simulink model "RM3_hwil2c_PI_test_desalv6"  (R2024a)
settings: Solver=ode45  StartTime=0  StopTime=387.2983  FixedStep=0.0005  MaxStep=0.0005  RelTol=1e-3
PreLoadFcn:
  | ng=150;
  | I_cont_design;
  | S_cont_design;
  | Theta_initial=Initial_Angle_Solver(simu_slr,simu_sll,simu_sll);
  | Wave_Analysis_WEC_Sim;
InitFcn:
  | %%% Hydraulic parameters
  | tsim = 1.5;
  | tc = 0.5;
  | Tss = 100e-6;
  | Nseg = 100;
  | Lpipe = 25;
  | Ps_high = 10e5;
  | Ps_low = 0*(Ps_high/3);
  | 
  | %%% Motor parameters
  | Pmax = 15e3;
  | Tmax = 50;
  | Teff = Tmax/2;
  | neff = 1500;
  | wref = 2000*(2*pi/60);
  | 
  | eff = 90;
  | Jmot = 0.005*5;
  | cd = 0.001;
  | kiw = 1e3/10;
  | kpw = 1e3/10;
  | udc = 250;
  | tr = 0.5;
values from neighbouring files (symbols this model uses):
  E_in = 42    [I_cont_design.m]
  In = 8    [I_cont_design.m]
  kii = kci    [I_cont_design.m]
  kis = kcs    [S_cont_design.m]
  kpi = kci/wzi    [I_cont_design.m]
  kps = kcs/wzs    [S_cont_design.m]
  kt = 0.091    [S_cont_design.m]
  La = 1.3e-3    (= 0.0013)    [I_cont_design.m]
  Nn = 4000    [S_cont_design.m]
  Ra = 0.7    [I_cont_design.m]
  simu = simulationClass()    [wecSimInputFile.m]
  simu_sll = 7    [wecSimInputFile.m]
  simu_slr = 1.5    [wecSimInputFile.m]
  T1_s = T1_s-TS    [Wave_Analysis_WEC_Sim.m]
  Ts = simu.dt    [I_cont_design.m]
  waves = waveClass('irregular')    [wecSimInputFile.m]
  wpi = wci*Kboosti    [I_cont_design.m]
  wps = wcs*Kboosts    [S_cont_design.m]
undefined symbols (not defined in the file or in its folder): body, constraint, geometry, hydroData, mooring, pn_flag, pto, T_s, Tf, Tt, Vf, Vfd, X, Y, Z
libraries: nesl_utility x43, fl_lib x25, sm_lib x23, WECSim_Lib_Body_Elements x9, WECSim_Lib_Constraints x5, sh_lib x3, spsMeanLib x2, spsSeriesRLCBranchLib x2, simulink x2, spsVoltageMeasurementLib x2, spsChopperLib x1, slpidlib x1
(part 1 of 5)
Description:
  | Segmented Pipeline Test Rig
  | 
  | The purpose of the rig is to investigate the water hammer effect, which takes place
  | when a variable orifice is abruptly shut off with full flow rate flowing through the
  | branch. The pressure sensor displays pressure at the orifice inlet, while
  | the flow rate meter shows flow rate through the branch. The water hammer-
  | like behavior of the pipeline can be investigated by changing pipeline
  | dimensions, number of segments in the pipeline model, fluid properties, and
  | valve closure speed and value.
  | 
  | 
  | Copyright 2008-2011 The MathWorks, Inc.
settings Model: SimulationMode=accelerator  Creator=MathWorks  LastModifiedBy=jniffene
settings SolverCC: NumberNewtonIterations=2  MaxConsecutiveMinStep=5  ZeroCrossControl=DisableAll  ZeroCrossAlgorithm=Adaptive  AlgebraicLoopSolver=TrustRegion  AutoInsertRateTranBlk=on
settings DataIOCC: LimitDataPoints=on  SaveFormat=Array  SignalLoggingSaveFormat=ModelDataLogs  ReturnWorkspaceOutputs=off
settings OptimizationCC: ExpressionDepthLimit=2147483647  InitFltsAndDblsToZero=on  EfficientMapNaN2IntZero=off  LifeSpan=inf  SimCompilerOptimization=on
settings DebuggingCC: SaveWithParameterizedLinksMsg=none  MergeDetectMultiDrivingBlocksExec=none  SignalResolutionControl=TryResolveAllWithWarning  IgnoredZcDiagnostic=none  SolverPrmCheckMsg=warning  MultiTaskDSMMsg=warning  MultiTaskCondExecSysMsg=none  FcnCallInpInsideContextMsg=warning  UnconnectedInputMsg=warning  UnconnectedOutputMsg=warning  UnconnectedLineMsg=warning  StateNameClashWarn=warning  SFUnexpectedBacktrackingDiag=warning  SFNoUnconditionalDefaultTransitionDiag=warning  ArithmeticOperatorsInVariantConditions=warning
settings HardwareCC: ProdBitPerPointer=32  ProdBitPerSizeT=32  ProdBitPerPtrDiffT=32  ProdLargestAtomicFloat=None  ProdIntDivRoundTo=Undefined  ProdEndianess=Unspecified  ProdWordSize=32  ProdHWDeviceType=32-bit Generic
settings ModelReferenceCC: EnableRefExpFcnMdlSchedulingChecks=on  PropagateSignalLabelsOutOfModel=off
settings SFSimCC: SimUseLocalCustomCode=off  CustomCodeUndefinedFunction=UseInterfaceOnly
settings RTWCC: RTWUseLocalCustomCode=off  GPUComputeCapability=3.5
settings CodeAppCC: StateflowObjectComments=on
settings GRTTargetCC: TargetFcnLib=ansi_tfl_tmw.mat  TargetLangStandard=C89/C90 (ANSI)  CombineOutputUpdateFcns=off  GRTInterface=on
settings ConfigComp: CovMetricSettings=dw  CovSaveCumulativeToWorkspaceVar=on  CovSaveSingleToWorkspaceVar=on  CovExternalEMLEnable=off  CovSFcnEnable=off
settings SimscapeCC: SimscapeNormalizeSystem=off  SimscapeLogType=local  SimscapeLogLimitData=off
settings ExplorerConfigSet: SimMechanicsOpenEditorOnUpdate=off

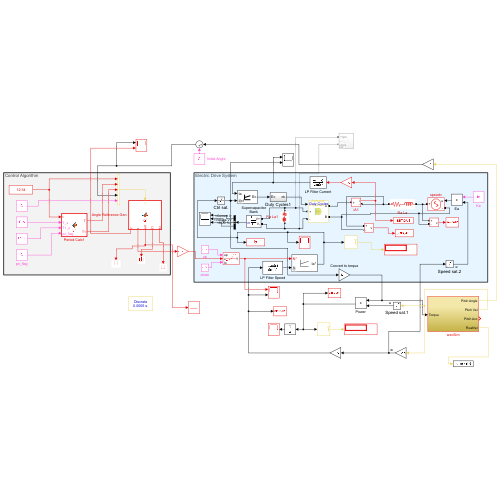
[thumbnail: Simulink's stored preview of the top-level diagram]
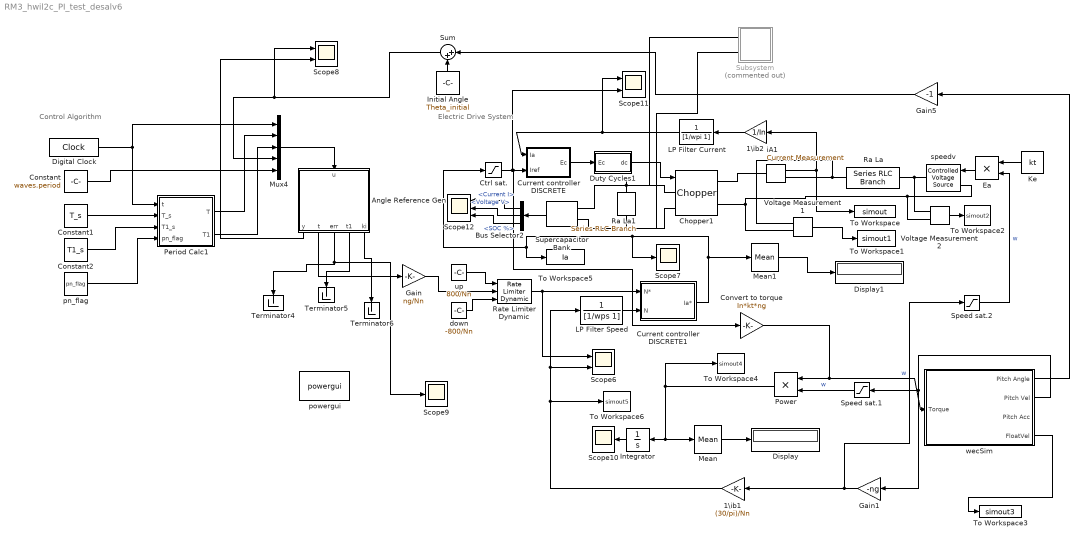
== system RM3_hwil2c_PI_test_desalv6 ==
  note: Electric Drive System
  note: Control Algorithm
  1\ib1 : Gain  Gain=(30/pi)/Nn  SaturateOnIntegerOverflow=on  OutDataTypeStr=Inherit: Same as input  ParamDataTypeStr=Inherit: Same as input
  1\ib2 : Gain  Gain=1/In  SaturateOnIntegerOverflow=on  OutDataTypeStr=Inherit: Same as input  ParamDataTypeStr=Inherit: Same as input
  Angle Reference Gen : MATLAB Function  TreatAsAtomicUnit=on
  Bus Selector2 : BusSelector  OutputSignals=Current I,Voltage V,SOC %
  Chopper1 : spsChopperLib/Chopper  detailLevel=Average  numQuad=4  SnubberResistance=Rsnb  SnubberCapacitance=Csnb  Ron=Ron  ForwardVoltages=[Vf,Vfd]  IGBTParameters=[Tf,Tt]  Ts=simu.dt  converterType=Inverter
      link override Chopper/Average_4q/Bus Selector: OutputSignals=IGBT 1&4
      settings: LibrarySourceBlock=electricdrivelib/Fundamental Drive Blocks/Chopper
  Constant : Constant  Value=waves.period
  Constant1 : Constant  Value=T_s
  Constant2 : Constant  Value=T1_s
  Convert to torque : Gain  Priority=1  Gain=In*kt*ng  SaturateOnIntegerOverflow=on  OutDataTypeStr=Inherit: Same as input  ParamDataTypeStr=Inherit: Same as input
  Ctrl sat. : Saturate  UpperLimit=2  LowerLimit=-2
  Current controller DISCRETE : Subsystem  mask(PI controller){Kp=kpi, Ki=kii, Ts=simu.dt}
      mask prompts: Kp "Proportional gain (Kp)"; Ki "Integral gain (Ki)"; Ts "Sample time (s) :"
      mask help: Proportional-Integral Speed Controller
      mask Display: plot(0,0,100,100,[35,35,65],[70,30,30],[35,65],[45,60])
  Current controller DISCRETE1 : Subsystem  mask(PI controller){Kp=kps*10, Ki=kis/60, Ts=Ts, Kd=0.05*3}
      mask prompts: Kp "Proportional gain (Kp)"; Ki "Integral gain (Ki)"; Ts "Sample time (s) :"; Kd "Differential gain (Kd)"
      mask help: Proportional-Integral Speed Controller
      mask Display: plot(0,0,100,100,[35,35,65],[70,30,30],[35,65],[45,60])
  Digital Clock : DigitalClock  SampleTime=simu.dt
  Display : Display
  Display1 : Display
  Duty Cycles1 : Subsystem
  Ea : Product
  Gain : Gain  Gain=ng/Nn
  Gain1 : Gain  Gain=-ng
  Gain5 : Gain  Gain=-1
  Initial Angle : Constant  Value=Theta_initial
  Integrator : Integrator
  Ke : Constant  Value=kt
  LP Filter Current : TransferFcn  Denominator=[1/wpi 1]
  LP Filter Speed : TransferFcn  Denominator=[1/wps 1]
  Mean : spsMeanLib/Mean  Freq=1/(4*waves.period)  Vinit=0  Ts=0
  Mean1 : spsMeanLib/Mean  Freq=1/(4*waves.period)  Vinit=0  Ts=0
  Mux4 : Mux  Inputs=5
  Period Calc1 : MATLAB Function  TreatAsAtomicUnit=on
  Power : Product
  Ra La : spsSeriesRLCBranchLib/Series RLC Branch  LConnTagsString=__new0  RConnTagsString=__new0  BranchType=RL  Resistance=Ra  Inductance=La  SetiL0=off  InitialCurrent=0  Capacitance=[]  Setx0=off  InitialVoltage=0  Measurements=None
  Ra La1 : spsSeriesRLCBranchLib/Series RLC Branch  LConnTagsString=__new0  RConnTagsString=__new0  BranchType=RL  Resistance=50  Inductance=0  SetiL0=off  InitialCurrent=0  Capacitance=[]  Setx0=off  InitialVoltage=0  Measurements=None
  Rate Limiter Dynamic : simulink/Discontinuities/Rate Limiter Dynamic
  Scope10 : Scope
  Scope11 : Scope  NumInputPorts=2
  Scope12 : Scope  NumInputPorts=3
  Scope6 : Scope  NumInputPorts=2
  Scope7 : Scope
  Scope8 : Scope  NumInputPorts=2
  Scope9 : Scope
  Speed sat.1 : Saturate  UpperLimit=(Nn*pi/30)/ng  LowerLimit=(-Nn*pi/30)/ng
  Speed sat.2 : Saturate  UpperLimit=(Nn*pi/30)  LowerLimit=(-Nn*pi/30)
  Subsystem : Subsystem  Commented=on
  Sum : Sum  Inputs=|++
  Supercapacitor Bank : spsSupercapacitorLib/Supercapacitor  C=100  Rdc=2e-3  Voltage=E_in  Ns=18  Np=1  Vinit=E_in  Temp=25  PresetModel=on  EstParam=off  Nc=1  r=1e-9  epsilon=6.0208e-10  Ich=10  Vstern="[0.161  2.7  7.8]"  Self_dis=on  Ioc=10  Vself="[48  47.8  47.06  44.65]"  demandeplot=off  I="[10  20 100  500]"  Units=sec  Vmax=0  If=0  deltaV=0  alpha=0  sec=0
      settings: LibrarySourceBlock=electricdrivelib/Extra Sources/Supercapacitor
  Terminator4 : Terminator
  Terminator5 : Terminator
  Terminator6 : Terminator
  To Workspace : ToWorkspace  VariableName=simout  SaveFormat=Timeseries  SampleTime=-1
  To Workspace1 : ToWorkspace  VariableName=simout1  SaveFormat=Timeseries  SampleTime=-1
  To Workspace2 : ToWorkspace  VariableName=simout2  SaveFormat=Timeseries  SampleTime=-1
  To Workspace3 : ToWorkspace  VariableName=simout3  SaveFormat=Timeseries  SampleTime=-1
  To Workspace4 : ToWorkspace  VariableName=simout4  SaveFormat=Timeseries  SampleTime=-1
  To Workspace5 : ToWorkspace  VariableName=Ia  SaveFormat=Timeseries  SampleTime=-1
  To Workspace6 : ToWorkspace  VariableName=simout5  SaveFormat=Timeseries  SampleTime=-1
  Voltage Measurement1 : spsVoltageMeasurementLib/Voltage Measurement  Tag=PoWeRsYsTeMmEaSuReMeNt  PhasorSimulation=off  OutputType=Magnitude  PSBequivalent=0
  Voltage Measurement2 : spsVoltageMeasurementLib/Voltage Measurement  Tag=PoWeRsYsTeMmEaSuReMeNt  PhasorSimulation=off  OutputType=Magnitude  PSBequivalent=0
  down : Constant  Value=-800/Nn
  iA1 : spsCurrentMeasurementLib/Current Measurement  PhasorSimulation=off  OutputType=Magnitude  PSBequivalent=0
  pn_flag : Constant  Value=pn_flag
  powergui : sps_lib/powergui  Priority=1  SimulationMode=Discrete  SampleTime=simu.dt  frequency=60  Iterations=50  frequencyindice=0  Pbase=100e6  ErrMax=1e-4  UnitsV=kV  UnitsW=MW  buscounter=0  FunctionMessages=off  echomessages=off  EnableUseOfTLC=off  CurrentSourceSwitches=off  DisableSnubberDevices=off  DisableRonSwitches=off  DisableVfSwitches=off  DisplayEquations=off  AutomaticDiscreteSolvers=off  SolverType=Tustin/Backward Euler (TBE)  Interpol=off  ExternalGateDelay=off  methode=off  Ts=10  x0status=blocks  SPID=off  SwTol=0  HookPort=off  NonlinearTolerance=1e-4  nMaxIteration=100  ContinueOnMaxIteration=off  RestoreLinks=warning  ResistiveCurrentMeasurement=off  Frange=[0:2:500]  Ylog=off  Xlog=on  ShowGrid=off  save=off  variable=ZData  structure=0  ZoomFFT=off  StartTime=0.0  cycles=1  DisplayStyle=1  fundamental=60  FreqAxis=off  MaxFrequency=1000  frequencyindicesteady=1  RmsSteady=1  display=off
  speedv : spsControlledVoltageSourceLib/Controlled Voltage Source  Description=source block  Initialize=on  Source_Type=AC  Amplitude=0  Phase=0  Frequency=0  Measurements=None
  up : Constant  Value=800/Nn
  wecSim : Subsystem
  wires:
  Mean1/1 -> Display1/1
  wecSim/4(FloatVel) -> To Workspace3/1
  Supercapacitor Bank/1 -> Bus Selector2/1
  Bus Selector2/1 -> Scope12/1  "<Current I>"
  iA1/1 -> 1\ib2/1, To Workspace/1
  LP Filter Current/1 -> Scope11/1, Current controller DISCRETE/1(Ia)
  Bus Selector2/3 -> Scope12/3  "<SOC %>"
  Bus Selector2/2 -> Scope12/2  "<Voltage V>"
  1\ib2/1 -> LP Filter Current/1
  wecSim/2(Pitch Vel) -> Speed sat.1/1, Gain1/1
  Angle Reference Gen/3(err) -> Scope9/1, Terminator4/1
  Speed sat.2/1 -> Ea/2  "w"
  1\ib1/1 -> To Workspace6/1, Scope6/2, LP Filter Speed/1
  Current controller DISCRETE/1(Ec) -> Duty Cycles1/1(Ec)
  Power/1 -> To Workspace4/1, Mean/1, Integrator/1
  Voltage Measurement2/1 -> To Workspace2/1
  pn_flag/1 -> Period Calc1/4(pn_flag)
  Duty Cycles1/1(dc) -> Chopper1/1
  Ctrl sat./1 -> Convert to torque/1, Current controller DISCRETE/2(Iref), Scope11/2
  Mean/1 -> Display/1
  Integrator/1 -> Scope10/1
  Current controller DISCRETE1/1(Ia*) -> Mean1/1, Scope7/1, To Workspace5/1, Ctrl sat./1
  Voltage Measurement1/1 -> To Workspace1/1
  Ea/1 -> speedv/1
  Angle Reference Gen/2(t) -> Gain/1
  Ke/1 -> Ea/1
  up/1 -> Rate Limiter Dynamic/1
  Rate Limiter Dynamic/1 -> Scope6/1, Current controller DISCRETE1/1(N*)
  Sum/1 -> Scope8/1, Mux4/4
  Mux4/1 -> Angle Reference Gen/1(u)
  Gain/1 -> Rate Limiter Dynamic/2
  Convert to torque/1 -> wecSim/1(Torque), Power/1
  Period Calc1/1(T) -> Mux4/2
  Gain1/1 -> Speed sat.2/1, 1\ib1/1  "w"
  down/1 -> Rate Limiter Dynamic/3
  LP Filter Speed/1 -> Current controller DISCRETE1/2(N)
  Digital Clock/1 -> Period Calc1/1(t), Mux4/1
  Initial Angle/1 -> Sum/2
  Angle Reference Gen/1(y) -> Scope8/2
  Constant/1 -> Mux4/5
  Angle Reference Gen/4(t1) -> Terminator5/1
  Constant2/1 -> Period Calc1/3(T1_s)
  Gain5/1 -> Sum/1
  Angle Reference Gen/5(ki) -> Terminator6/1
  wecSim/1(Pitch Angle) -> Gain5/1
  Constant1/1 -> Period Calc1/2(T_s)
  Period Calc1/2(T1) -> Mux4/3
  Speed sat.1/1 -> Power/2  "w"
  connections:
  Voltage Measurement1/LConn2 -- speedv/LConn1 -- Voltage Measurement2/LConn2 -- Chopper1/RConn2
  Voltage Measurement2/LConn1 -- Ra La/RConn1 -- speedv/RConn1
  Voltage Measurement1/LConn1 -- Ra La/LConn1 -- iA1/RConn1
  Chopper1/RConn1 -- iA1/LConn1
  Subsystem/LConn2 -- Chopper1/LConn2 -- Ra La1/RConn1 -- Supercapacitor Bank/LConn2
  Subsystem/LConn1 -- Chopper1/LConn1 -- Ra La1/LConn1 -- Supercapacitor Bank/LConn1

== system RM3_hwil2c_PI_test_desalv6/Current controller DISCRETE ==
  Ia : Inport
  Iref : Inport  Port=2
  Ctrl sat. : Saturate  UpperLimit=1  LowerLimit=-1
  Integral gain : Gain  Gain=Ki  SaturateOnIntegerOverflow=on  OutDataTypeStr=Inherit: Same as input  ParamDataTypeStr=Inherit: Same as input
  Integrator : Integrator
  Proportional gain : Gain  Gain=Kp  SaturateOnIntegerOverflow=on  OutDataTypeStr=Inherit: Same as input  ParamDataTypeStr=Inherit: Same as input
  Sum1 : Sum  Inputs=-+  InputSameDT=on  SaturateOnIntegerOverflow=on  OutDataTypeStr=Inherit: Same as first input
  Sum2 : Sum  InputSameDT=on  SaturateOnIntegerOverflow=on  OutDataTypeStr=Inherit: Same as first input
  Ec : Outport  InitialOutput=0
  wires:
  Ctrl sat./1 -> Ec/1
  Sum2/1 -> Ctrl sat./1
  Integrator/1 -> Sum2/2
  Iref/1 -> Sum1/2
  Ia/1 -> Sum1/1
  Sum1/1 -> Proportional gain/1, Integral gain/1
  Integral gain/1 -> Integrator/1
  Proportional gain/1 -> Sum2/1

== system RM3_hwil2c_PI_test_desalv6/Current controller DISCRETE1 ==
  N* : Inport
  N : Inport  Port=2
  Discrete PID Controller : slpidlib/PID Controller  Controller=PID  Form=Parallel  TimeDomain=Continuous-time  UseExternalTs=off  SampleTime=-1  IntegratorMethod=Trapezoidal  FilterMethod=Trapezoidal  ControllerParametersSource=internal  P=Kp  I=Ki  UseKiTs=off  D=Kd  UseExternalDerivativeSource=off  N=100  UseFilter=on  TunerSelectOption=Transfer Function Based (PID Tuner App)  InitialConditionSource=internal  InitialConditionForIntegrator=0  InitialConditionForFilter=0  DifferentiatorICPrevScaledInput=0  ExternalReset=none  TrackingMode=off  Kt=1  LimitOutput=off  SatLimitsSource=internal  UpperSaturationLimit=2  LowerSaturationLimit=-2  LinearizeAsGain=off  AntiWindupMode=none  Kb=1  LimitIntegrator=off  UpperIntegratorSaturationLimit=inf  LowerIntegratorSaturationLimit=-inf  POutMin=[]  POutMax=[]  IOutMin=[]  IOutMax=[]  DOutMin=[]  DOutMax=[]  NOutMin=[]  NOutMax=[]  SumOutMin=[]  SumOutMax=[]  SaturationOutMin=[]  SaturationOutMax=[]  PParamMin=[]  PParamMax=[]  IParamMin=[]  IParamMax=[]  DParamMin=[]  DParamMax=[]  NParamMin=[]  NParamMax=[]  KbParamMin=[]  KbParamMax=[]  KtParamMin=[]  KtParamMax=[]  KbOutMin=[]  KbOutMax=[]  KtOutMin=[]  KtOutMax=[]  IntegratorOutMin=[]  IntegratorOutMax=[]  FilterOutMin=[]  FilterOutMax=[]  SumI1OutMin=[]  SumI1OutMax=[]  SumI2OutMin=[]  SumI2OutMax=[]  SumI3OutMin=[]  SumI3OutMax=[]  SumI4OutMin=[]  SumI4OutMax=[]  SumDOutMin=[]  SumDOutMax=[]  DifferentiatorOutMin=[]  DifferentiatorOutMax=[]  FilterDiffOutCoefMin=[]  FilterDiffOutCoefMax=[]  ReciprocalOutMin=[]  ReciprocalOutMax=[]  SumDenOutMin=[]  SumDenOutMax=[]  SumNumOutMin=[]  SumNumOutMax=[]  DivideOutMin=[]  DivideOutMax=[]  UdiffTsProdOutMin=[]  UdiffTsProdOutMax=[]  NTsProdOutMin=[]  NTsProdOutMax=[]  UintegralTsProdOutMin=[]  UintegralTsProdOutMax=[]  UngainTsProdOutMin=[]  UngainTsProdOutMax=[]  ClampingZeroOutDataTypeStr=Inherit: Inherit via back propagation  ClampingZeroOutMin=[]  ClampingZeroOutMax=[]  FilterDenConstantOutDataTypeStr=Inherit: Inherit via back propagation  FilterDenConstantOutMin=[]  FilterDenConstantOutMax=[]  PCopyOutDataTypeStr=Inherit: Inherit via back propagation  PCopyOutMin=[]  PCopyOutMax=[]  NCopyOutDataTypeStr=Inherit: Inherit via back propagation  NCopyOutMin=[]  NCopyOutMax=[]  IntegratorContinuousStateAttributes=''  IntegratorStateMustResolveToSignalObject=off  IntegratorRTWStateStorageClass=Auto  FilterContinuousStateAttributes=''  FilterStateMustResolveToSignalObject=off  FilterRTWStateStorageClass=Auto  ParallelPVariant=InternalParameters  IdealPVariant=Disabled  IVariant=InternalParameters  DVariant=InternalParameters  IntegratorVariant=Continuous  SatVariant=Disabled  AWVariant=Passthrough  PCopyVariant=Disabled  TRVariant=Disabled  FdbkBlocksVariant=Forward  IdealPFdbkVariant=Disabled  SatFdbkVariant=Disabled  DerivativeFilterVariant=ContFilter  NVariant=InternalParameters  NCopyVariant=Disabled  FilterICVariant=InternalICsFilter  IntegratorICVariant=InternalICs  ExternalResetVariant=Disabled  TRSumVariant=Passthrough  SumFdbkVariant=Disabled  SumVariant=Sum_PID  TsampFilterVariant=InternalTs  TsampNgainVariant=Passthrough  TsampIntegralVariant=Disabled_SignalSpec  ExternalSaturationOutDataTypeStr=Inherit: Same as second input  DerivativeSourceVariant=ErrorSignal
  Sum1 : Sum  Inputs=+-  InputSameDT=on  SaturateOnIntegerOverflow=on  OutDataTypeStr=Inherit: Same as first input
  Ia* : Outport  InitialOutput=0
  wires:
  Discrete PID Controller/1 -> Ia*/1
  N/1 -> Sum1/2
  N*/1 -> Sum1/1
  Sum1/1 -> Discrete PID Controller/1

== system RM3_hwil2c_PI_test_desalv6/Duty Cycles1 ==
  Ec : Inport
  Add : Sum  Inputs=+-
  Bus Creator2 : BusCreator  Inputs=2
  Constant : Constant
  Duty Cycle : Fcn  Expr=0.5*(u[1]+1)
  dc : Outport
  wires:
  Bus Creator2/1 -> dc/1
  Ec/1 -> Duty Cycle/1
  Constant/1 -> Add/1
  Duty Cycle/1 -> Add/2, Bus Creator2/1  "IGBT 1&4"
  Add/1 -> Bus Creator2/2  "IGBT 2&3"

== system RM3_hwil2c_PI_test_desalv6/Subsystem ==
  note: Copyright 2016 - 2020 MathWorks AB
  "Brine " : fl_lib/Hydraulic/Hydraulic Elements/Hydraulic Reference
  Clock1 : Clock
  Current-Voltage Simscape Interface : spsCurrentVoltageSimscapeInterfaceLib/Current-Voltage Simscape Interface  DFT=on  FMode=Low pass filter (continuous)  T=1e-6  Ts=50e-6  i0=0  v0=E_in  Sd=Specialized Power Systems side  Measurements=off
      settings: LibrarySourceBlock=|
      | sps_lib/Utilities/Current-Voltage
      | Simscape Interface
  Electrical Reference : fl_lib/Electrical/Electrical Elements/Electrical Reference
  Fixed-Displacement Pump : sh_lib/Pumps and Motors/Fixed-Displacement Pump  D=(5e-6)/100 m^3/rad  loss_spec=1  w_nominal=188 rad/s  pr_nominal=100e5 Pa  visc_nominal=18 cSt  dens_nominal=984.328 kg/m^3  efficiency_vol=1  no_load_torque=0 N*m  torque_pressure_coeff=1*(5e-6)*((1)/(1)-1 ) N*m/Pa  p_diff_eff_TLU=[100000.0, 1000000.0, 2000000.0] Pa  omega_eff_TLU=[25.0, 50.0, 100.0, 200.0, 300.0, 400.0] rad/s  vol_eff_TLU=[0.816, 0.908, 0.954, 0.977, 0.981, 0.984; 0.325, 0.663, 0.831, 0.916, 0.925, 0.946; 0.137, 0.568, 0.78, 0.892, 0.893, 0.91]  mech_eff_TLU=[0.996, 0.996, 0.996, 0.996, 0.996, 0.996; 0.988, 0.989, 0.989, 0.989, 0.989, 0.99; 0.981, 0.981, 0.982, 0.982, 0.983, 0.984]  p_diff_loss_TLU=[100000.0, 1000000.0, 2000000.0] Pa  omega_loss_TLU=[25.0, 50.0, 100.0, 200.0, 300.0, 400.0] rad/s  vol_loss_TLU=[0.023, 0.023, 0.023, 0.023, 0.0285, 0.032; 0.0844, 0.0842, 0.0845, 0.084, 0.1125, 0.108; 0.1079, 0.108, 0.11, 0.108, 0.1605, 0.18] * 1e-3 m^3/s  mech_loss_TLU=[0.002, 0.002, 0.002, 0.002, 0.002, 0.002; 0.0607, 0.0556, 0.0556, 0.0556, 0.0556, 0.0505; 0.1937, 0.1937, 0.1833, 0.1833, 0.1729, 0.1626] N*m  pressure_threshold=1e5 Pa  omega_threshold=10 rad/s  quadrant_check=0  pressure_check=0  min_valid_pressure=0 Pa  vol_eff_min=1e-3  vol_eff_max=1  mech_eff_min=1e-3  mech_eff_max=1
      settings: InternalSimscapePortConfiguration="{\"Bottom\":[],\"Left\":[{\"id\":\"S\",\"label\":\"S\",\"type\":\"foundation.mechanical.rotational.rotational\"}],\"Right\":[{\"id\":\"P\",\"label\":\"P\",\"type\":\"foundation.hydraulic.hydraulic\"},{\"id\":\"T\",\"label\":\"T\",\"type\":\"foundation.hydraulic.hydraulic\"}],\"Top\":[]}"
  HR2 : fl_lib/Hydraulic/Hydraulic Elements/Hydraulic Reference  Tag=Factory Generic
  Hydraulic Fluid : sh_lib/Hydraulic Utilities/Hydraulic Fluid  Tag=Factory Generic  SelFluid=24  SysTemp=60  TrapAir=0.001  ViscDerFactor=1  range_error=2
  Logging : Subsystem
  Mechanical Rotational Reference : fl_lib/Mechanical/Rotational Elements/Mechanical Rotational Reference
  Motor : ee_lib/Electromechanical/Motor & Drive (System Level)  torque_speed_param=2  overtorque_param=ee.enum.electromech.overtorque.no  T_t=[0.09 0.08 0.07 0] N*m  T_t_intermittent=[.36, .32, .28, 0] N*m  T_t_2D=[.09, .09, .09; .08, .08, .08; .07, .07, .07; 0, 0, 0] N*m  T_t_intermittent_2D=[.36, .36, .36; .32, .32, .32; .28, .28, .28; 0, 0, 0] N*m  w_t=[ 0 3.75e+3 7.5e+3 8e+3 ] rpm  vdc_t=[6, 12, 24] V  torque_max=5 N*m  power_max=100 W  torque_max_intermittent=0.4 N*m  power_max_intermittent=120 W  time_overtorque=30 s  time_recover=60 s  Tc=0.05 s  EnableSwitch=simscape.enum.onoff.off  losses_param=1  eff=eff  w_eff=neff rpm  T_eff=Teff N*m  Piron=0 W  Pbase=0 W  w_eff_vec=[-8000 -4000 0 4000 8000] rpm  T_eff_vec=[0 0.03 0.06 0.09] N*m  v_eff_vec=[100, 250, 400] V  losses_mat=[1.49 1.67 2.21 3.10; 0.42 0.69 1.14 2.03; 0.06 0.24 0.78 1.68; 0.42 0.69 1.14 2.03; 1.49 1.67 2.21 3.10] W  efficiency_mat=[95, 95, 95, 95; 95, 95, 95, 95; 95, 95, 95, 95; 95, 95, 95, 95; 95, 95, 95, 95]  losses_mat_3D=ones(5, 4, 3) W  efficiency_mat_3D=95 * ones(5, 4, 3)  Res=0 Ohm  enable_fault=simscape.enum.onoff.off  fault_condition=1  fault_threshold=0.5  J=4.2e-4 kg*m^2  lam=1.5e-4 N*m/(rad/s)  speed0=0 rpm  faulted_specify=off  faulted_priority=None  faulted=0  faulted_nominal_specify=off  faulted_nominal_value=1  faulted_nominal_unit=1  isSwitchedOff_specify=off  isSwitchedOff_priority=None  isSwitchedOff=0  isSwitchedOff_nominal_specify=off  isSwitchedOff_nominal_value=1  isSwitchedOff_nominal_unit=1  torqueLimitContinuous_specify=off  torqueLimitContinuous_priority=None  torqueLimitContinuous=0 N*m  torqueLimitContinuous_nominal_specify=off  torqueLimitContinuous_nominal_value=1  torqueLimitContinuous_nominal_unit=N*m  alpha=3.93e-3 1/K  Tmeas=25 degC  Tmeas2=125 degC  losses_mat_T2=[1.49, 1.74, 2.49, 3.74; .42, .67, 1.42, 2.67; .06, .31, 1.06, 2.31; .42, .67, 1.42, 2.67; 1.49, 1.74, 2.49, 3.74] W  efficiency_mat_T2=[95, 95, 95, 95; 95, 95, 95, 95; 95, 95, 95, 95; 95, 95, 95, 95; 95, 95, 95, 95]  losses_mat_3D_T2=ones(5, 4, 3) W  efficiency_mat_3D_T2=95 * ones(5, 4, 3)  thermal_mass=100 J/K  initial_temperature=25 degC
      settings: LogSimulationData=on
  Permeate : fl_lib/Hydraulic/Hydraulic Elements/Hydraulic Reference
  Q_sensor_vfd : Subsystem
  RO Membrane : Subsystem
      mask Display: image('/Users/yyu/Dropbox/WorksNREL/ResearchWork/Desalination/JSME Runs/Images/ReverseOsmosisMembrane.jpg');
  Sensor : Subsystem
  Sensor Mec (VFD) : Subsystem
  Simulink-PS Converter1 : nesl_utility/Simulink-PS Converter  PhysicalDomain=network_engine_domain  SubClassName=ps_input  LeftPortType=input  RightPortType=output  PseudoPeriodic=off  Frequencies=[]  NoiseDistribution=none  NoiseParameters=[]  Unit=rad/s  AffineConversion=off  FilteringAndDerivatives=zero  SimscapeFilterOrder=1  InputFilterTimeConstant=.001  UdotUserProvided=1
  Solver Configuration : nesl_utility/Solver Configuration  PhysicalDomain=network_engine_domain  SubClassName=solver  LeftPortType=input  RightPortType=generic  Tones=[]  Harmonics=[]  SimulateNoise=off  Profile=off  UseLocalSampling=off  EnableSwitchedLinearOptims=on  FrequencyDomain=off  UseCCode=off  RelTol=0.001  AbsTol=1e-06  MinStep=1e-09  ToWorkspace=off  RevertToSquareIcSolve=off  NumHomotopyIterations=100  PhasorMode=off  PhasorModeNumHarmonics=1  ConsistencySolver=NEWTON_FTOL  IndexReductionMethod=DerivativeReplacement  DoDC=off  ResidualTolerance=1e-9  ConsistencyTolSource=GLOBAL  ConsistencyAbsTol=0.001  ConsistencyRelTol=0.001  ConsistencyTolFactor=0.001  UseLocalSolver=off  LocalSolverChoice=NE_BACKWARD_EULER_ADVANCER  ResolveIndetEquations=on  FunctionEvalNumThread=1  LocalSolverSampleTime=Tss  DoFixedCost=off  MaxNonlinIter=3  MaxModeIter=2  ComputeImpulses=off  ImpulseIterations=2  LinearAlgebra=Sparse  LinearAlgebraNumThread=0  EquationFormulation=NE_TIME_EF  DelaysMemoryBudget=1024  AutomaticFiltering=on  FilteringTimeConstant=0.001  PartitionStorageMethod=AS_NEEDED  PartitionMemoryBudget=1024  PartitionMethod=FAST  MultibodyUseLocalSolver=off  MultibodyLocalSolverChoice=ODE1  MultibodyLocalSolverSampleTime=0.001
  Speed control : Subsystem
  speed profile : Lookup_n-D  NumberOfTableDimensions=1  BreakpointsForDimension1=[0 10 20]  Table=[0 1 1]*1.122790000000000e+02  InternalRulePriority=Speed  RndMeth=Simplest
  +sps : PMIOPort  Side=Left
  -sps : PMIOPort  Port=2  Side=Left
  wires:
  Clock1/1 -> speed profile/1
  speed profile/1 -> Simulink-PS Converter1/1
  connections:
  Electrical Reference/LConn1 -- Current-Voltage Simscape Interface/RConn2 -- Motor/RConn1
  Fixed-Displacement Pump/LConn1 -- Sensor Mec (VFD)/RConn1
  "Brine "/LConn1 -- RO Membrane/RConn2
  Solver Configuration/RConn1 -- Fixed-Displacement Pump/RConn1 -- Hydraulic Fluid/RConn1 -- Q_sensor_vfd/LConn1
  Simulink-PS Converter1/RConn1 -- Speed control/LConn1
  Speed control/RConn1 -- Motor/LConn2
  Motor/RConn2 -- Speed control/LConn2
  Permeate/LConn1 -- RO Membrane/RConn1
  Current-Voltage Simscape Interface/RConn1 -- Sensor/LConn1
  Q_sensor_vfd/RConn1 -- RO Membrane/LConn1
  Sensor/RConn1 -- Motor/LConn1
  Motor/LConn3 -- Sensor Mec (VFD)/LConn1
  Fixed-Displacement Pump/RConn2 -- HR2/LConn1
  Motor/RConn3 -- Mechanical Rotational Reference/LConn1
  Current-Voltage Simscape Interface/LConn2 -- -sps/RConn1
  Current-Voltage Simscape Interface/LConn1 -- +sps/RConn1

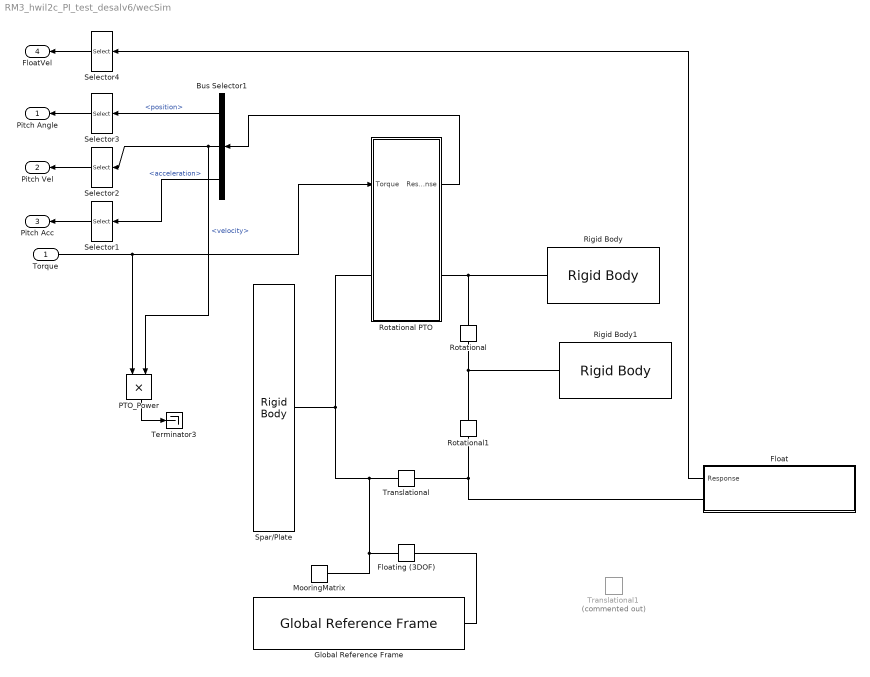
== system RM3_hwil2c_PI_test_desalv6/wecSim ==
  Torque : Inport
  Bus Selector1 : BusSelector  OutputSignals=position,velocity,acceleration
  Float : Subsystem  AncestorBlock=WECSim_Lib_Body_Elements/Rigid Body  Variant=on  AllowZeroVariantControls=on  mask(Rigid Body){body=body(1), InputFileText=Global Reference Frame option "Use Input File" is selected., h5File=hydroData/*.h5, geometryFile=geometry/*.stl, mass=0, inertia=0 0 0, inertiaProducts=0 0 0, nonHydro=0, nonlinearHydro=0, centerGravity=0 0 0, centerBuoyancy=0 0 0, dof=6, volume=0, QTFs=0, flex=0, displacement=0 0 0, axis=0 1 0, angle=0, option=0, cd=0 0 0, ca=0 0 0, area=0 0 0, VME=0, rgME=0 0 0, z=0 0 1}
      mask prompts: body "Body Number:"; mass "Body Mass [kg]:"; inertia "MoI [kg*m^2]:"; inertiaProducts "Product of Inertia [kg*m^2]"; nonHydro "Nonhydro Body"; nonlinearHydro "Nonlinear Hydrodynamics"; centerGravity "Center of gravity [m]"; centerBuoyancy "Center of buoyancy [m]"; dof "Degrees of freedom"; volume "Displaced Volume [m^3]"; flex "Flexible Body"; displacement "Initial Linear Displacement"; axis "Initial Angular Displacement Axis"; angle "Initial Angular Displacement"; option "On/Off"; cd "Drag coefficient"; ca "Added mass coefficient"; area "Characteristic Area"; VME "Characteristic Volume"; rgME "Point of Application"; z "Z axis"
      mask help:
      | A rigid body has no generalized body modes. It can be a standard hydrodynamic body, a drag body, or a non-hydrodynamic body.
      |
      | The variable name input below must be 'body(i)' where i=1,2,...
      | body(i) must be defined in the input file with the fields appropriate to each variant.
      mask init:
      | if exist('body','var')
      |     %%
      |     % Hydro Body
      |     h = [gcb '/Hydrodynamic Body'];
      |     responseName = ['sv_b' num2str(body.number) '_hydroBody'];
      |     set_param(h,'VariantControl',responseName);
      |     %%
      |     % Hydro Body Morison Element: Off
      |     h = [gcb '/Hydrodynamic Body/Morison Element and Viscous Damping Force Calculation/Morison Element Variant Subsystem/Morison Element Off'];
      |     responseName = ['sv_b' num2str(body.number) '_MEOff'];
      |     set_param(h,'VariantControl',responseName);
      |     %%
      |     % Hydro Body Morison Element: On
      |     h = [gcb '/Hydrodynamic Body/Morison Element and Viscous Damping Force Calculation/Morison Element Variant Subsystem/Morison Element On'];
      |     responseName = ['sv_b' num2str(body.number) '_MEOn'];
      |     set_param(h,'VariantControl',responseName);
      |     %%
      |     % Hydro Body Nonlinear Froude Krylov Force: Off
      |     h = [gcb '/Hydrodynamic Body/Wave Diffraction and Excitation Force Calculation/Nonlinear FK Force Variant Subsystem/No Nonlinear FroudeKrylov Force'];
      |     responseName = ['sv_b' num2str(body.number) '_linearHydro'];
      |     set_param(h,'VariantControl',responseName);
      |     %%
      |     % Hydro Body Nonlinear Froude Krylov Force: On
      |     h = [gcb '/Hydrodynamic Body/Wave Diffraction and Excitation Force Calculation/Nonlinear FK Force Variant Subsystem/With Nonlinear FroudeKrylov Force'];
      |     responseName = ['sv_b' num2str(body.number) '_nonlinearHydro'];
      |     set_param(h,'VariantControl',responseName);
      |     %%
      |     % Hydro Body Nonlinear Restoring: Off
      |     h = [gcb '/Hydrodynamic Body/Hydrostatic Restoring Force Calculation/Linear and Nonlinear Restoring Force Variant Subsystem/Linear Hydrostatic Restoring Force'];
      |     responseName = ['sv_b' num2str(body.number) '_linearHydro'];
      |     set_param(h,'VariantControl',responseName);
      |     %%
      |     % Hydro Body Nonlinear Restoring: On
      |     h = [gcb '/Hydrodynamic Body/Hydrostatic Restoring Force Calculation/Linear and Nonlinear Restoring Force Variant Subsystem/Nonlinear Hydrostatic Restoring Force'];
      |     responseName = ['sv_b' num2str(body.number) '_nonlinearHydro'];
      |     set_param(h,'VariantControl',responseName);
      |     %%
      |     % Hydro Body Regular Excitation Passive Yaw: Off
      |     h = [gcb '/Hydrodynamic Body/Wave Diffraction and Excitation Force Calculation/Linear Wave Excitation Force Variant Subsystem/Regular Wave ' newline 'Excitation Force'];
      |     responseName = ['sv_regularWaves_b' num2str(body.number)];
      |     set_param(h,'VariantControl',responseName);
      |     %%
      |     % Hydro Body Regular Excitation Passive Yaw: On
      |     h = [gcb '/Hydrodynamic Body/Wave Diffraction and Excitation Force Calculation/Linear Wave Excitation Force Variant Subsystem/Regular Wave ' newline 'NonLinear Yaw'];
      |     responseName = ['sv_regularWavesYaw_b' num2str(body.number)];
      |     set_param(h,'VariantControl',responseName);
      |     %%    
      |     % Hydro Body Irregular Excitation Passive Yaw: Off
      |     h = [gcb '/Hydrodynamic Body/Wave Diffraction and Excitation Force Calculation/Linear Wave Excitation Force Variant Subsystem/Irregular Wave ' newline 'Excitation Force'];
      |     responseName = ['sv_irregularWaves_b' num2str(body.number)];
      |     set_param(h,'VariantControl',responseName);
      |     %%
      |     % Hydro Body Irregular Excitation Passive Yaw: On
      |     h = [gcb '/Hydrodynamic Body/Wave Diffraction and Excitation Force Calculation/Linear Wave Excitation Force Variant Subsystem/Irregular Wave ' newline 'NonLinearYaw'];
      |     responseName = ['sv_irregularWavesYaw_b' num2str(body.number)];
      |     set_param(h,'VariantControl',responseName);
      |     %%
      |     % Hydro Body Nonlinear Froude Krylov or Restoring: Instantaneous Free Surface
      |     h = [gcb '/Hydrodynamic Body/Nonlinear Wave Elevation/Linear or Instantaneous Free Surface/Instantaneous Water Free Surface'];
      |     responseName = ['sv_b' num2str(body.number) '_instFS'];
      |     set_param(h,'VariantControl',responseName);
      |     %%
      |     % Hydro Body Nonlinear Froude Krylov or Restoring: Mean Free Surface
      |     h = [gcb '/Hydrodynamic Body/Nonlinear Wave Elevation/Linear or Instantaneous Free Surface/Mean Water Free Surface'];
      |     responseName = ['sv_b' num2str(body.number) '_meanFS'];
      |     set_param(h,'VariantControl',responseName);
      |     %% Variable hydro on/off
      |     % Variable hydro control - variable hydro off
      |     h = [gcb '/Hydrodynamic Body/Variable Hydrodynamics Control/Variable Hydrodynamics Subsystem/noVariableHydro'];
      |     responseName = ['sv_b' num2str(body.number) '_noVariableHydro'];
      |     set_param(h,'VariantControl',responseName);
      |     % Variable hydro control - variable hydro on
      |     h = [gcb '/Hydrodynamic Body/Variable Hydrodynamics Control/Variable Hydrodynamics Subsystem/variableHydro'];
      |     responseName = ['sv_b' num2str(body.number) '_variableHydro'];
      |     set_param(h,'VariantControl',responseName);
      |     % CIC - variable hydro off
      |     h = [gcb '/Hydrodynamic Body/Wave Radiation Forces Calculation/SS CI and Constant-Damping-CoeVariant Subsystem/Convolution Integral Calculation/Convolution Variant Subsystem/Convolution Integral Calculation'];
      |     responseName = ['sv_b' num2str(body.number) '_noVariableHydro'];
      |     set_param(h,'VariantControl',responseName);
      |     % CIC - variable hydro on
      |     h = [gcb '/Hydrodynamic Body/Wave Radiation Forces Calculation/SS CI and Constant-Damping-CoeVariant Subsystem/Convolution Integral Calculation/Convolution Variant Subsystem/Convolution Integral Surface Calculation'];
      |     responseName = ['sv_b' num2str(body.number) '_variableHydro'];
      |     set_param(h,'VariantControl',responseName);
      |     %%
      |     % Non-Hydro Body
      |     h = [gcb '/Non-Hydro Body'];
      |     responseName = ['sv_b' num2str(body.number) '_nonHydroBody'];
      |     set_param(h,'VariantControl',responseName);
      |     %%
      |     % Drag Body
      |     h = [gcb '/Drag Body'];
      |     responseName = ['sv_b' num2str(body.number) '_dragBody'];
      |     set_param(h,'VariantControl',responseName);
      |     %%
      |     % Drag Body Morison Element: Off
      |     h = [gcb '/Drag Body/Morison Element and Viscous Damping Force Calculation/Morison Element Variant Subsystem/Morison Element Off'];
      |     responseName = ['sv_b' num2str(body.number) '_MEOff'];
      |     set_param(h,'VariantControl',responseName);
      |     %%
      |     % Drag Body Morison Element: On
      |     h = [gcb '/Drag Body/Morison Element and Viscous Damping Force Calculation/Morison Element Variant Subsystem/Morison Element On'];
      |     responseName = ['sv_b' num2str(body.number) '_MEOn'];
      |     set_param(h,'VariantControl',responseName);
      |     %% 
      |     % Hydro Body QTF: Off
      |     h = [gcb '/Hydrodynamic Body/Wave Diffraction and Excitation Force Calculation/Second Order Excitation Force Variant Subsystem/No Second Order Excitation Force'];
      |     responseName = ['sv_b' num2str(body.number) '_noSecondOrderExt'];
      |     set_param(h,'VariantControl',responseName);
      |     %%
      |     % Hydro Body QTF: On
      |     h = [gcb '/Hydrodynamic Body/Wave Diffraction and Excitation Force Calculation/Second Order Excitation Force Variant Subsystem/With Second Order Excitation Force'];
      |     responseName = ['sv_b' num2str(body.number) '_secondOrderExt'];
      |     set_param(h,'VariantControl',responseName);
      |     %%
      |     % Set zero active variant controls to prevent label issue
      |     set_param(gcb,'AllowZeroVariantControls','on');
      | end
      | clear bc h geomFile responseName
      settings: AttributesFormatString=%<body>
      mask Help:
      | A rigid body has no generalized body modes. It can be a standard hydrodynamic body, a drag body, or a non-hydrodynamic body.
      | 
      | The variable name input below must be 'body(i)' where i=1,2,...
      | body(i) must be defined in the input file with the fields appropriate to each variant.
      mask TypeOptions nonHydro: 0 | 1 | 2
      mask Callback nonHydro: bodyClassCallback(gcbh)
      mask TypeOptions nonlinearHydro: 0 | 1 | 2
      mask TypeOptions QTFs: 0 | 1 | 2
      mask TypeOptions flex: 0 | 1
      mask TypeOptions option: 0 | 1 | 2
      mask Callback option: bodyClassCallback(gcbh)
      mask DialogControl CustomParameterGroup Prompt: Custom Parameters
      mask DialogControl std_opts Prompt: Standard Options
      mask DialogControl H5button Prompt: Select .h5 File
      mask DialogControl H5button Callback: h5ButtonCallback(gcbh)
      mask DialogControl STLbutton Prompt: Select .stl File
      mask DialogControl STLbutton Callback: stlButtonCallback(gcbh)
      mask DialogControl inertia Tooltip: Moment of Inertia
      mask DialogControl inertiaProducts Tooltip: Product of Inertia (Ixy, Ixz, Iyz)
      mask DialogControl initial Prompt: Initial Displacement
      mask DialogControl morisonElement Prompt: Morison Element
      mask DialogControl rgME Tooltip: The vector from the body COG to point of application for the Morison Element
      mask DialogControl z Tooltip: The unit normal vector center axis of the Morison Element
  Floating (3DOF) : WECSim_Lib_Constraints/Floating (3DOF)  constraint=constraint(1)  loc="0  0  0"  displacement=0 0 0  y=0 1 0  z=0 0 1  upperLimitSpecify=off  upperLimitBound=0  upperLimitTransitionRegionWidth=0  upperLimitStiffness=0  upperLimitDamping=0  lowerLimitSpecify=off  lowerLimitBound=0  lowerLimitTransitionRegionWidth=0  lowerLimitStiffness=0  lowerLimitDamping=0
      settings: AttributesFormatString=%<constraint>  SourceProductName=WEC-Sim
  Global Reference Frame : WECSim_Lib_Frames/Global Reference Frame  waves=waves  simu=simu  InputMethod=Input File  InputFile=wecSimInputFile.m  mode=normal  explorer=off  solver=ode4  startTime=0  rampTime=100  endTime=400  dt=0.1  cicEndTime=60  stateSpace=0  WaveClass=regular  height=2.5  period=8  elevationFile=NOT DEFINED  spectrumFile=NOT DEFINED  direction=0  spread=1  spectrumType=NOT DEFINED  phaseSeed=0  option=EqualEnergy
  MooringMatrix : WECSim_Lib_Moorings/MooringMatrix  mooring=mooring(1)  loc=0 0 0  preTension=[0 0 0 0 0 0]  stiffness={ '0', '0', '0', '0', '0', '0'; '0', '0', '0', '0', '0', '0'; '0', '0', '0', '0', '0', '0'; '0', '0', '0', '0', '0', '0'; '0', '0', '0', '0', '0', '0'; '0', '0', '0', '0', '0', '0' }  damping={ '0', '0', '0', '0', '0', '0'; '0', '0', '0', '0', '0', '0'; '0', '0', '0', '0', '0', '0'; '0', '0', '0', '0', '0', '0'; '0', '0', '0', '0', '0', '0'; '0', '0', '0', '0', '0', '0' }
      settings: AttributesFormatString=%<mooring>  SourceProductName=WEC-Sim
  PTO_Power : Product  Inputs=**
  Rigid Body : WECSim_Lib_Body_Elements/Rigid Body  body=body(3)  h5File=hydroData/*.h5  geometryFile=geometry/*.stl  mass=0  inertia=0 0 0  inertiaProducts=0 0 0  nonHydro=0  nonlinearHydro=0  centerGravity=0 0 0  centerBuoyancy=0 0 0  dof=6  volume=0  QTFs=0  displacement=0 0 0  axis=0 1 0  angle=0  option=0  cd=0 0 0  ca=0 0 0  area=0 0 0  VME=0  rgME=0 0 0  z=0 0 1
      link override Non-Hydro Body/Mass: Value=body.mass
  Rigid Body1 : WECSim_Lib_Body_Elements/Rigid Body  body=body(4)  h5File=hydroData/*.h5  geometryFile=geometry/*.stl  mass=0  inertia=0 0 0  inertiaProducts=0 0 0  nonHydro=0  nonlinearHydro=0  centerGravity=0 0 0  centerBuoyancy=0 0 0  dof=6  volume=0  QTFs=0  displacement=0 0 0  axis=0 1 0  angle=0  option=0  cd=0 0 0  ca=0 0 0  area=0 0 0  VME=0  rgME=0 0 0  z=0 0 1
      link override Non-Hydro Body/Mass: Value=body.mass
  Rotational : WECSim_Lib_Constraints/Rotational  constraint=constraint(3)  loc="0  0  0"  displacement=0 0 0  y=0 1 0  z=0 0 1  upperLimitSpecify=off  upperLimitBound=0  upperLimitTransitionRegionWidth=0  upperLimitStiffness=0  upperLimitDamping=0  lowerLimitSpecify=off  lowerLimitBound=0  lowerLimitTransitionRegionWidth=0  lowerLimitStiffness=0  lowerLimitDamping=0
      settings: AttributesFormatString=%<constraint>
  Rotational PTO : Subsystem  AncestorBlock=WECSim_Lib_PTOs/Rotational PTO  mask(PTO){pto=pto(1), InputFileText=Global Reference Frame option "Use Input File" is selected., loc=0  0  0, stiffness=0, damping=0, equilibriumPosition=0, pretension=0, displacement=0 0 0, x=, y=0 1 0, z=0 0 1, upperLimitSpecify=off, upperLimitBound=0, upperLimitTransitionRegionWidth=0, upperLimitStiffness=0, upperLimitDamping=0, lowerLimitSpecify=off, lowerLimitBound=0, lowerLimitTransitionRegionWidth=0, lowerLimitStiffness=0, lowerLimitDamping=0}
      mask prompts: pto "PTO Name:"; loc "Location [m]:"; stiffness "Stiffness [N/m]:"; damping "Damping [N/(m/s)]:"; equilibriumPosition "Equilibrium position [m, deg]:"; pretension "Pretension [N, Nm]:"; displacement "Initial linear displacement [m]:"; x "X-axis [m]:"; y "Y-axis [m]:"; z "Z-axis [m]:"; upperLimitSpecify "Upper limit"; upperLimitBound "Upper limit bound [m, deg]:"; upperLimitTransitionRegionWidth "Upper limit transition region width [m, deg]:"; upperLimitStiffness "Upper limit stiffness [N/m, Nm/rad]:"; upperLimitDamping "Upper limit damping [N/(m/s), Nm/(rad/s)]:"; lowerLimitSpecify "Lower limit"; lowerLimitBound "Upper limit bound [m, deg]:"; lowerLimitTransitionRegionWidth "Upper limit transition region width [m, deg]:"; lowerLimitStiffness "Upper limit stiffness [N/m, Nm/rad]:"; lowerLimitDamping "Upper limit damping [N/(m/s), Nm/(rad/s)]:"
      mask help:
      | Constrains the follower to rotational motion relative to the base, about
      | the PTO's Y-direction and adds PTO stiffness and damping.
      |
      | The variable name input below must be 'pto(i)' where i=1,2,...
      | pto(i) must be defined in the input file with the following fields:
      |
      |     .name (required)
      |             String.
      |             PTO name. Must comply with Matlab's variable naming rules.
      |     .location (required)
      |             3x1 vector [x y z] in meters.
      |             PTO location. Default = [0 0 0]
      |     .stiffness (optional)
      |             Float.
      |             PTO linear spring stiffness. Default = 0
      |     .damping (optional)
      |             Float.
      |             PTO linear damping coefficient. Default = 0
      |     .orientation.z (optional)
      |             3x1 vector [x y z].
      |             Direction of the PTO's Z-coordinate. Default = [0 0 1]
      |     .orientation.y (optional)
      |             3x1 vector [x y z].
      |             Direction of the PTO's Y-coordinate. Default = [0 1 0]
      mask init:
      | if exist('pto','var')
      |     h=[gcb '/To Workspace'];
      |     responseName=['pto' num2str(pto.number) '_out'];
      |     set_param(h,'VariableName',responseName);
      |     h=[gcb '/Pitch PCC ' newline '(Revolute Joint)'];
      |     try % this should catch any version issue for which these parameters do not exist
      |         set_param(h,'upperLimitSpecify',pto.hardStops.upperLimitSpecify)
      |         set_param(h,'lowerLimitSpecify',pto.hardStops.lowerLimitSpecify)
      |     end
      |     if pto.extension.PositionTargetSpecify == 1
      |         set_param(h,'PositionTargetSpecify','on')
      |     else
      |         set_param(h,'PositionTargetSpecify','off')
      |     end
      | end
      | 
      | pto.checkLoc('E');
      settings: AttributesFormatString=%<pto>
      mask Help:
      | Constrains the follower to rotational motion relative to the base, about
      | the PTO's Y-direction and adds PTO stiffness and damping.
      | 
      | The variable name input below must be 'pto(i)' where i=1,2,...
      | pto(i) must be defined in the input file with the following fields:
      | 
      |     .name (required)
      |             String.
      |             PTO name. Must comply with Matlab's variable naming rules.
      |     .location (required)
      |             3x1 vector [x y z] in meters.
      |             PTO location. Default = [0 0 0]
      |     .stiffness (optional)
      |             Float.
      |             PTO linear spring stiffness. Default = 0
      |     .damping (optional)
      |             Float.
      |             PTO linear damping coefficient. Default = 0
      |     .orientation.z (optional)
      |             3x1 vector [x y z].
      |             Direction of the PTO's Z-coordinate. Default = [0 0 1]
      |     .orientation.y (optional)
      |             3x1 vector [x y z].
      |             Direction of the PTO's Y-coordinate. Default = [0 1 0]
      mask Callback upperLimitSpecify: hardStopCallback(gcbh)
      mask Callback lowerLimitSpecify: hardStopCallback(gcbh)
      mask DialogControl InputFileGroup Prompt: Input File
      mask DialogControl CustomParameterGroup Prompt: Custom Parameters
      mask DialogControl std_opts Prompt: Standard options
      mask DialogControl orientations Prompt: Orientation
      mask DialogControl x Tooltip: This axis is defined by the y and z axes.
      mask DialogControl Container7 Prompt: Hard Stop
  Rotational1 : WECSim_Lib_Constraints/Rotational  constraint=constraint(4)  loc="0  0  0"  displacement=0 0 0  y=0 1 0  z=0 0 1  upperLimitSpecify=off  upperLimitBound=0  upperLimitTransitionRegionWidth=0  upperLimitStiffness=0  upperLimitDamping=0  lowerLimitSpecify=off  lowerLimitBound=0  lowerLimitTransitionRegionWidth=0  lowerLimitStiffness=0  lowerLimitDamping=0
      settings: AttributesFormatString=%<constraint>
  Selector1 : Selector  InputPortWidth=6  IndexOptions=Index vector (dialog)  Indices=5  OutputSizes=1
  Selector2 : Selector  InputPortWidth=6  IndexOptions=Index vector (dialog)  Indices=5  OutputSizes=1
  Selector3 : Selector  InputPortWidth=6  IndexOptions=Index vector (dialog)  Indices=5  OutputSizes=1
  Selector4 : Selector  InputPortWidth=6  IndexOptions=Index vector (dialog)  Indices=3  OutputSizes=1
  Spar/Plate : WECSim_Lib_Body_Elements/Rigid Body  body=body(2)  h5File=hydroData/*.h5  geometryFile=geometry/*.stl  mass=0  inertia=0 0 0  inertiaProducts=0 0 0  nonHydro=0  nonlinearHydro=0  centerGravity=0 0 0  centerBuoyancy=0 0 0  dof=6  volume=0  QTFs=0  displacement=0 0 0  axis=0 1 0  angle=0  option=0  cd=0 0 0  ca=0 0 0  area=0 0 0  VME=0  rgME=0 0 0  z=0 0 1
  Terminator3 : Terminator
  Translational : WECSim_Lib_Constraints/Translational  constraint=constraint(2)  loc="0  0  0"  displacement=0 0 0  y=0 1 0  z=0 0 1  upperLimitSpecify=off  upperLimitBound=0  upperLimitTransitionRegionWidth=0  upperLimitStiffness=0  upperLimitDamping=0  lowerLimitSpecify=off  lowerLimitBound=0  lowerLimitTransitionRegionWidth=0  lowerLimitStiffness=0  lowerLimitDamping=0
      settings: AttributesFormatString=%<constraint>
  Translational1 : WECSim_Lib_Constraints/Translational  Commented=on  constraint=constraint(1)  loc="0  0  0"  displacement=0 0 0  y=0 1 0  z=0 0 1  upperLimitSpecify=off  upperLimitBound=0  upperLimitTransitionRegionWidth=0  upperLimitStiffness=0  upperLimitDamping=0  lowerLimitSpecify=off  lowerLimitBound=0  lowerLimitTransitionRegionWidth=0  lowerLimitStiffness=0  lowerLimitDamping=0
      settings: AttributesFormatString=%<constraint>  SourceProductName=WEC-Sim
  Pitch Angle : Outport
  Pitch Vel : Outport  Port=2
  Pitch Acc : Outport  Port=3
  FloatVel : Outport  Port=4
  wires:
  PTO_Power/1 -> Terminator3/1
  Bus Selector1/1 -> Selector3/1  "<position>"
  Rotational PTO/1(Response) -> Bus Selector1/1
  Bus Selector1/2 -> PTO_Power/2, Selector2/1  "<velocity>"
  Selector1/1 -> Pitch Acc/1
  Selector2/1 -> Pitch Vel/1
  Selector3/1 -> Pitch Angle/1
  Bus Selector1/3 -> Selector1/1  "<acceleration>"
  Torque/1 -> Rotational PTO/1(Torque), PTO_Power/1
  Float/1(Response) -> Selector4/1
  Selector4/1 -> FloatVel/1
  connections:
  Translational/RConn1 -- Rotational1/LConn1 -- Float/RConn1
  Rigid Body/RConn1 -- Rotational/RConn1 -- Rotational PTO/RConn1
  Rotational/LConn1 -- Rotational1/RConn1 -- Rigid Body1/RConn1
  Floating (3DOF)/LConn1 -- MooringMatrix/LConn1 -- Translational/LConn1 -- Rotational PTO/LConn1 -- Spar/Plate/RConn1
  Floating (3DOF)/RConn1 -- Global Reference Frame/RConn1

== system RM3_hwil2c_PI_test_desalv6/Subsystem/Logging ==
  Mux1 : Mux  Inputs=6
  To Workspace2 : ToWorkspace  VariableName=simout7  SaveFormat=Structure With Time  SampleTime=0.01
  wires:
  [Permeate] -> Mux1/1
  Mux1/1 -> To Workspace2/1
  [To_RO] -> Mux1/2
  [Pressure] -> Mux1/3
  [Brine] -> Mux1/4
  [Pshaft_vfd] -> Mux1/5
  [Pmot] -> Mux1/6

== system RM3_hwil2c_PI_test_desalv6/Subsystem/Q_sensor_vfd ==
  Hydraulic Flow Rate Sensor : fl_lib/Hydraulic/Hydraulic Sensors/Hydraulic Flow Rate Sensor
  PS-Simulink Converter1 : nesl_utility/PS-Simulink Converter  PhysicalDomain=network_engine_domain  SubClassName=ps_output  LeftPortType=input  RightPortType=output  PseudoPeriodic=off  Frequencies=[]  VectorFormat=1-D array  Unit=1  AffineConversion=off
  in : PMIOPort  Side=Left
  ut : PMIOPort  Port=2  Side=Right
  tag scope: q_vfd=global
  wires:
  PS-Simulink Converter1/1 -> [q_vfd]
  connections:
  Hydraulic Flow Rate Sensor/LConn1 -- in/RConn1
  PS-Simulink Converter1/LConn1 -- Hydraulic Flow Rate Sensor/RConn1
  Hydraulic Flow Rate Sensor/RConn2 -- ut/RConn1
